simulink model "bicycleModel"  (R2020a)
settings: Solver=VariableStepAuto  StartTime=0.0  StopTime=40  RelTol=1e-3
undefined symbols (not defined in the file or in its folder): DiscIntNeverNeededParam
libraries: simulink x1
settings Model: Creator=usuario  LastModifiedBy=usuario

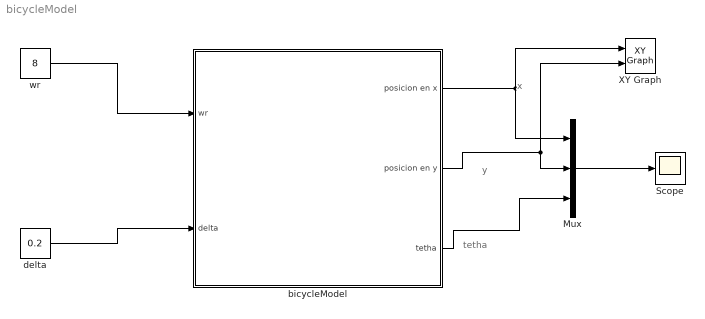
== system bicycleModel ==
  note: tetha
  note: y
  note: x
  Mux : Mux  Inputs=3
  Scope : Scope
  XY Graph : simulink/Sinks/XY Graph  xmin=-20  xmax=20  ymin=-20  ymax=20  st=-1
  bicycleModel : Subsystem  mask{sampleTime=0.01, inicialY=1, inicialX=1, tethaInicial=pi, wheelRadius=0.5, wheelBase=1.5}
      mask prompts: inicialY "posicion inicial Y"; inicialX "posicion inicial x"
      mask Display: image('C:\Users\usuario\Downloads\33066859-esta-es-una-ilustración-de-un-robot-en-la-bicicleta.jpg'); % Use "Edit Image" on toolstrip to change.
  delta : Constant  Value=0.2
  wr : Constant  Value=8
  wires:
  wr/1 -> bicycleModel/1(wr)
  delta/1 -> bicycleModel/2(delta)
  bicycleModel/1(posicion en x) -> Mux/1, XY Graph/1
  bicycleModel/2(posicion en y) -> Mux/2, XY Graph/2
  bicycleModel/3(tetha) -> Mux/3
  Mux/1 -> Scope/1

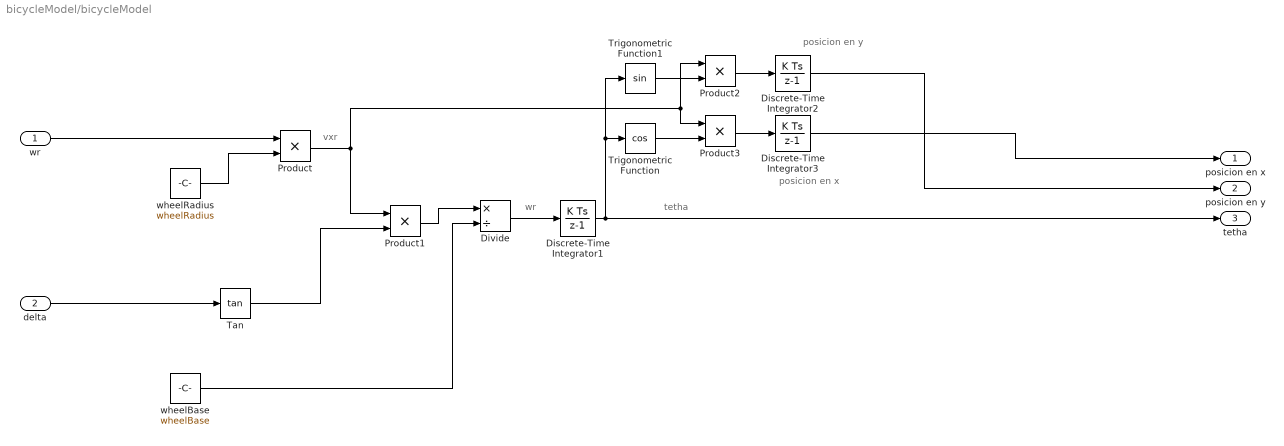
== system bicycleModel/bicycleModel ==
  note: tetha
  note: posicion en x
  note: posicion en y
  note: vxr
  note: wr
  wr : Inport
  delta : Inport  Port=2
  Discrete-Time Integrator1 : DiscreteIntegrator  InitialCondition=tethaInicial  SampleTime=sampleTime  ICPrevOutput=DiscIntNeverNeededParam  ICPrevScaledInput=DiscIntNeverNeededParam
  Discrete-Time Integrator2 : DiscreteIntegrator  InitialCondition=inicialY  SampleTime=sampleTime  ICPrevOutput=DiscIntNeverNeededParam  ICPrevScaledInput=DiscIntNeverNeededParam
  Discrete-Time Integrator3 : DiscreteIntegrator  InitialCondition=inicialX  SampleTime=sampleTime  ICPrevOutput=DiscIntNeverNeededParam  ICPrevScaledInput=DiscIntNeverNeededParam
  Divide : Product  Inputs=*/
  Product{,1..3} (4 alike) : Product
  Tan : Trigonometry  Operator=tan
  Trigonometric Function : Trigonometry  Operator=cos
  Trigonometric Function1 : Trigonometry
  wheelBase : Constant  Value=wheelBase
  wheelRadius : Constant  Value=wheelRadius
  posicion en x : Outport
  posicion en y : Outport  Port=2
  tetha : Outport  Port=3
  wires:
  Trigonometric Function1/1 -> Product2/2
  Discrete-Time Integrator1/1 -> tetha/1, Trigonometric Function1/1, Trigonometric Function/1
  Product2/1 -> Discrete-Time Integrator2/1
  Product1/1 -> Divide/1
  Product/1 -> Product1/1, Product2/1, Product3/1
  Tan/1 -> Product1/2
  Divide/1 -> Discrete-Time Integrator1/1
  Discrete-Time Integrator2/1 -> posicion en y/1
  wheelBase/1 -> Divide/2
  wheelRadius/1 -> Product/2
  Trigonometric Function/1 -> Product3/2
  Product3/1 -> Discrete-Time Integrator3/1
  Discrete-Time Integrator3/1 -> posicion en x/1
  wr/1 -> Product/1
  delta/1 -> Tan/1
